simulink model "Bai30"  (R2016a)
settings: Solver=VariableStepAuto  StartTime=0.0  StopTime=10.0  RelTol=1e-3
settings Model: Creator=0818562562  LastModifiedBy=0818562562

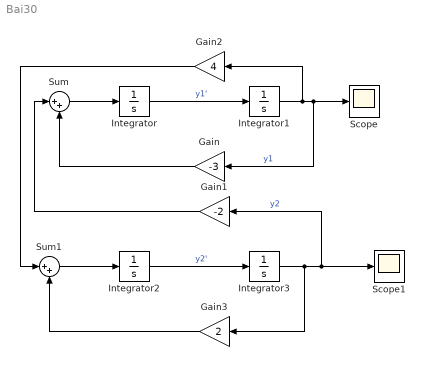
== system Bai30 ==
  Gain : Gain  Gain=-3
  Gain1 : Gain  Gain=-2
  Gain2 : Gain  Gain=4
  Gain3 : Gain  Gain=2
  Integrator : Integrator
  Integrator1 : Integrator  InitialCondition=1
  Integrator2 : Integrator
  Integrator3 : Integrator  InitialCondition=1
  Scope : Scope
  Scope1 : Scope
  Sum : Sum  Inputs=|++
  Sum1 : Sum  Inputs=|++
  wires:
  Integrator1/1 -> Gain2/1, Gain/1, Scope/1  "y1"
  Integrator/1 -> Integrator1/1  "y1'"
  Integrator3/1 -> Gain3/1, Gain1/1, Scope1/1  "y2"
  Integrator2/1 -> Integrator3/1  "y2'"
  Gain/1 -> Sum/2
  Gain1/1 -> Sum/1
  Sum/1 -> Integrator/1
  Gain3/1 -> Sum1/2
  Gain2/1 -> Sum1/1
  Sum1/1 -> Integrator2/1
